simulink model "v2_new_5d_Z1_PbhPin_sim"  (Simulink 7.8)
settings: Solver=ode15s  StartTime=0.0  StopTime=100000  MaxStep=1  MinStep=1e-12  RelTol=1e-10
values from neighbouring files (symbols this model uses):
  K = minreal(K)    [Hinf_Linear_Z1_Pbh.m]    (also in Hinf_MIMO_Linear_Z1_PinPt.m; Hinf_MIMO_Nonlinear_Z1_PbhPin.m; Hinf_MIMO_Nonlinear_Z1_PinPt.m; Hinf_MISO_Linear_Z1_PbhWin.m)
  u0 = [z1;z2;0;0]    [Hinf_Linear_Z1_Pbh.m]    (also in Hinf_MIMO_Linear_Z1_PinPt.m; Hinf_MIMO_Nonlinear_Z1_PbhPin.m; Hinf_MIMO_Nonlinear_Z1_PinPt.m; Hinf_MISO_Linear_Z1_PbhWin.m)
  y0 = v2_new_5d_model(0,x0,u0,'measurements',par)    [v2_new_5d_linmodl_num.m]
undefined symbols (not defined in the file or in its folder): Dd, Du
settings Model: Creator=jahansha  LastModifiedBy=matslie
settings DebuggingCC: FcnCallInpInsideContextMsg=Use local settings

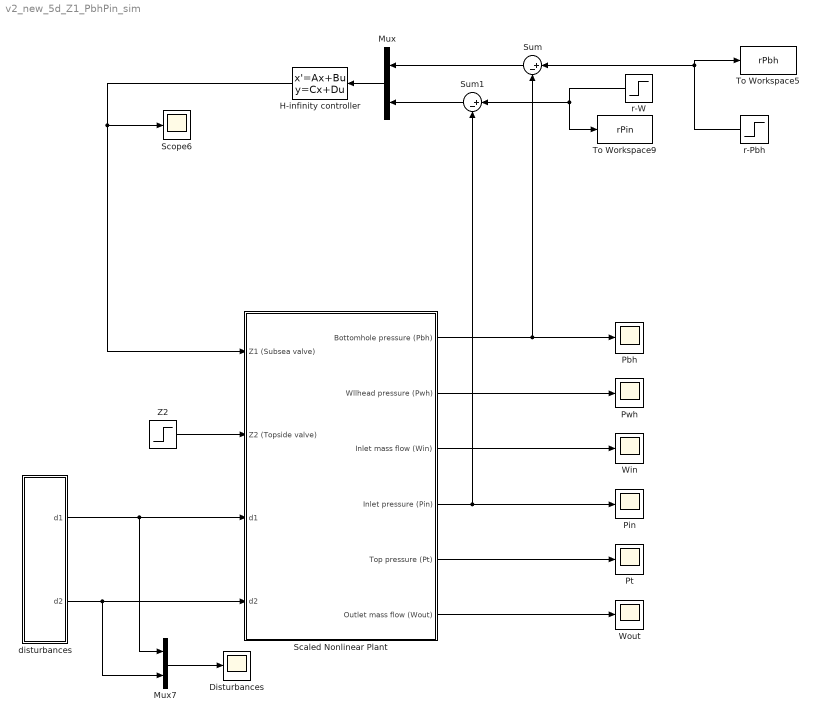
== system v2_new_5d_Z1_PbhPin_sim ==
  Disturbances : Scope
      settings: TimeRange=8000  YMin=1.38778e-017  YMax=0.275  SaveName=ScopeData5
  H-infinity controller : StateSpace  A=K.a  B=K.b  C=K.c  D=K.d
  Mux : Mux  Inputs=2
  Mux7 : Mux  Inputs=2
  Pbh : Scope
      settings: TimeRange=100000  YMin=-0.1915  YMax=-0.184  SaveName=ScopeData3
  Pin : Scope
      settings: TimeRange=8000  YMin=0.105  YMax=0.113  SaveName=ScopeData7
  Pt : Scope
      settings: TimeRange=8000  YMin=0.105  YMax=0.113
  Pwh : Scope
      settings: TimeRange=10000  YMin=-0.0275  YMax=-0.0075  SaveName=ScopeData4
  Scaled Nonlinear Plant : Subsystem
  Scope6 : Scope
      settings: TimeRange=8000  YMin=-8.5e+130  YMax=1e+130
  Sum : Sum  Inputs=|+-
  Sum1 : Sum  Inputs=|+-
  To Workspace5 : ToWorkspace  VariableName=rPbh  SampleTime=-1  SaveFormat=Array
  To Workspace9 : ToWorkspace  VariableName=rPin  SampleTime=-1  SaveFormat=Array
  Win : Scope
      settings: YMin=0.225  YMax=0.55  SaveName=ScopeData2
  Wout : Scope
      settings: TimeRange=100000  YMin=-0.6  YMax=1.4  SaveName=ScopeData6
  Z2 : Step  Time=0  After=0  SampleTime=0
  disturbances : Subsystem
  r-Pbh : Step  Time=100000  After=0  SampleTime=0
  r-W : Step  Time=10000  After=0  SampleTime=0
  wires:
  Mux7/1 -> Disturbances/1
  disturbances/1(d1) -> Mux7/1, Scaled Nonlinear Plant/3(d1)
  disturbances/2(d2) -> Mux7/2, Scaled Nonlinear Plant/4(d2)
  Scaled Nonlinear Plant/1(Bottomhole pressure (Pbh)) -> Pbh/1, Sum/2
  Scaled Nonlinear Plant/2(Wllhead pressure (Pwh)) -> Pwh/1
  Scaled Nonlinear Plant/3(Inlet mass flow (Win)) -> Win/1
  Scaled Nonlinear Plant/4(Inlet pressure (Pin)) -> Pin/1, Sum1/2
  Scaled Nonlinear Plant/5(Top pressure (Pt)) -> Pt/1
  r-Pbh/1 -> To Workspace5/1, Sum/1
  Mux/1 -> H-infinity controller/1
  r-W/1 -> To Workspace9/1, Sum1/1
  H-infinity controller/1 -> Scope6/1, Scaled Nonlinear Plant/1(Z1 (Subsea valve))
  Sum/1 -> Mux/1
  Sum1/1 -> Mux/2
  Scaled Nonlinear Plant/6(Outlet mass flow (Wout)) -> Wout/1
  Z2/1 -> Scaled Nonlinear Plant/2(Z2 (Topside valve))

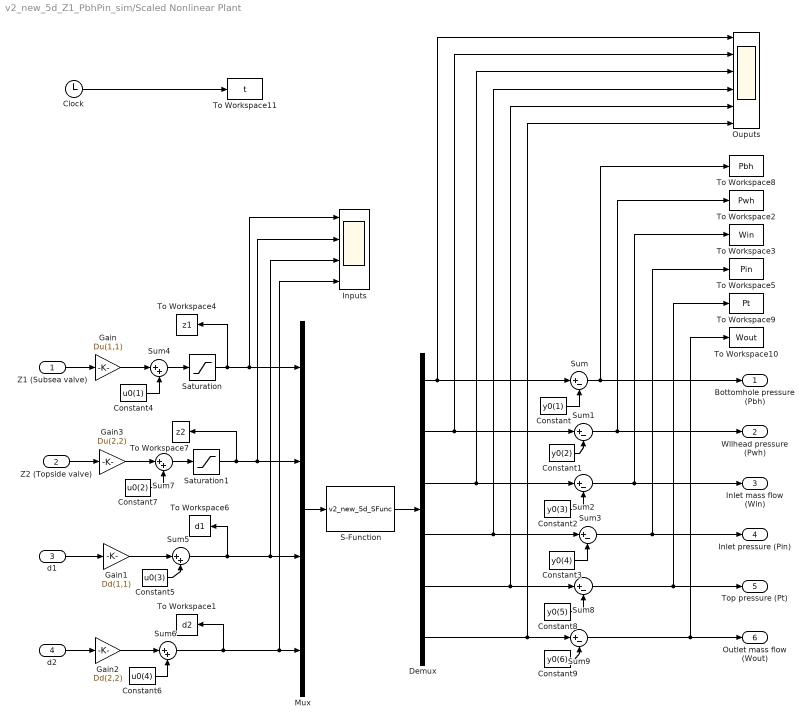
== system v2_new_5d_Z1_PbhPin_sim/Scaled Nonlinear Plant ==
  Z1 (Subsea valve) : Inport
  Z2 (Topside valve) : Inport  Port=2
  d1 : Inport  Port=3
  d2 : Inport  Port=4
  Clock : Clock
  Constant : Constant  Value=y0(1)
  Constant1 : Constant  Value=y0(2)
  Constant2 : Constant  Value=y0(3)
  Constant3 : Constant  Value=y0(4)
  Constant4 : Constant  Value=u0(1)
  Constant5 : Constant  Value=u0(3)
  Constant6 : Constant  Value=u0(4)
  Constant7 : Constant  Value=u0(2)
  Constant8 : Constant  Value=y0(5)
  Constant9 : Constant  Value=y0(6)
  Demux : Demux  Outputs=6
  Gain : Gain  Gain=Du(1,1)
  Gain1 : Gain  Gain=Dd(1,1)
  Gain2 : Gain  Gain=Dd(2,2)
  Gain3 : Gain  Gain=Du(2,2)
  Inputs : Scope  NumInputPorts=4
      settings: TimeRange=8000  YMin=-1~-5~-5~-5  YMax=1~5~5~5  SaveName=ScopeData9
  Mux : Mux
  Ouputs : Scope  NumInputPorts=6
      settings: TimeRange=100000  YMin=279.857~71.1957~11.0392~71.1306~51.6171~11.4892  YMax=279.857~71.1957~11.0392~71.1307~51.6171~11.4892  SaveName=ScopeData10
  S-Function : S-Function  FunctionName=v2_new_5d_SFunc  EnableBusSupport=off
  Saturation : Saturate  UpperLimit=1  LowerLimit=0
  Saturation1 : Saturate  UpperLimit=1  LowerLimit=0
  Sum{,1..3,8..9} (6 alike) : Sum  Inputs=|+-
  Sum{4..7} (4 alike) : Sum  Inputs=|++
  To Workspace1 : ToWorkspace  VariableName=d2  SampleTime=-1  SaveFormat=Array
  To Workspace10 : ToWorkspace  VariableName=Wout  SampleTime=-1  SaveFormat=Array
  To Workspace11 : ToWorkspace  VariableName=t  SampleTime=-1  SaveFormat=Array
  To Workspace2 : ToWorkspace  VariableName=Pwh  SampleTime=-1  SaveFormat=Array
  To Workspace3 : ToWorkspace  VariableName=Win  SampleTime=-1  SaveFormat=Array
  To Workspace4 : ToWorkspace  VariableName=z1  SampleTime=-1  SaveFormat=Array
  To Workspace5 : ToWorkspace  VariableName=Pin  SampleTime=-1  SaveFormat=Array
  To Workspace6 : ToWorkspace  VariableName=d1  SampleTime=-1  SaveFormat=Array
  To Workspace7 : ToWorkspace  VariableName=z2  SampleTime=-1  SaveFormat=Array
  To Workspace8 : ToWorkspace  VariableName=Pbh  SampleTime=-1  SaveFormat=Array
  To Workspace9 : ToWorkspace  VariableName=Pt  SampleTime=-1  SaveFormat=Array
  Bottomhole pressure (Pbh) : Outport
  Wllhead pressure (Pwh) : Outport  Port=2
  Inlet mass flow (Win) : Outport  Port=3
  Inlet pressure (Pin) : Outport  Port=4
  Top pressure (Pt) : Outport  Port=5
  Outlet mass flow (Wout) : Outport  Port=6
  wires:
  Mux/1 -> S-Function/1
  S-Function/1 -> Demux/1
  Demux/1 -> Sum/1, Ouputs/1
  Demux/2 -> Sum1/1, Ouputs/2
  Constant1/1 -> Sum1/2
  Demux/3 -> Ouputs/3, Sum2/1
  Constant3/1 -> Sum3/2
  Sum/1 -> Bottomhole pressure (Pbh)/1, To Workspace8/1
  Sum1/1 -> Wllhead pressure (Pwh)/1, To Workspace2/1
  Sum2/1 -> Inlet mass flow (Win)/1, To Workspace3/1
  Demux/4 -> Sum3/1, Ouputs/4
  Sum3/1 -> Inlet pressure (Pin)/1, To Workspace5/1
  Constant4/1 -> Sum4/2
  Z1 (Subsea valve)/1 -> Gain/1
  Gain/1 -> Sum4/1
  Constant5/1 -> Sum5/2
  Gain1/1 -> Sum5/1
  d1/1 -> Gain1/1
  Sum5/1 -> To Workspace6/1, Mux/3, Inputs/3
  Constant6/1 -> Sum6/2
  Gain2/1 -> Sum6/1
  d2/1 -> Gain2/1
  Sum6/1 -> To Workspace1/1, Mux/4, Inputs/4
  Saturation/1 -> Mux/1, To Workspace4/1, Inputs/1
  Sum4/1 -> Saturation/1
  Constant7/1 -> Sum7/2
  Z2 (Topside valve)/1 -> Gain3/1
  Gain3/1 -> Sum7/1
  Sum7/1 -> Saturation1/1
  Saturation1/1 -> To Workspace7/1, Mux/2, Inputs/2
  Constant8/1 -> Sum8/2
  Demux/5 -> Sum8/1, Ouputs/5
  Sum8/1 -> Top pressure (Pt)/1, To Workspace9/1
  Constant9/1 -> Sum9/2
  Demux/6 -> Sum9/1, Ouputs/6
  Sum9/1 -> Outlet mass flow (Wout)/1, To Workspace10/1
  Constant/1 -> Sum/2
  Constant2/1 -> Sum2/2
  Clock/1 -> To Workspace11/1

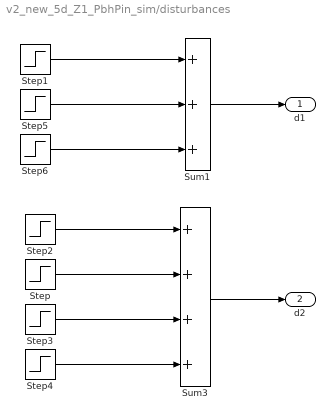
== system v2_new_5d_Z1_PbhPin_sim/disturbances ==
  Step : Step  Time=30000  After=-1  SampleTime=0
  Step1 : Step  Time=10000  SampleTime=0
  Step2 : Step  Time=20000  SampleTime=0
  Step3 : Step  Time=40000  After=-1  SampleTime=0
  Step4 : Step  Time=60000  SampleTime=0
  Step5 : Step  Time=50000  After=-1  SampleTime=0
  Step6 : Step  Time=70000  After=-1  SampleTime=0
  Sum1 : Sum  Inputs=+++
  Sum3 : Sum  Inputs=++++
  d1 : Outport
  d2 : Outport  Port=2
  wires:
  Step2/1 -> Sum3/1
  Step/1 -> Sum3/2
  Step3/1 -> Sum3/3
  Sum3/1 -> d2/1
  Step4/1 -> Sum3/4
  Step1/1 -> Sum1/1
  Step5/1 -> Sum1/2
  Sum1/1 -> d1/1
  Step6/1 -> Sum1/3
